simulink model "sampleModel337"  (R2021b)
settings: Solver=VariableStepAuto  StartTime=0.0  StopTime=10.0  RelTol=1e-3
undefined symbols (not defined in the file or in its folder): DiscIntNeverNeededParam, Newton, Raphson
libraries: simulink x14, slpidlib x1
settings Model: Creator=user  LastModifiedBy=user

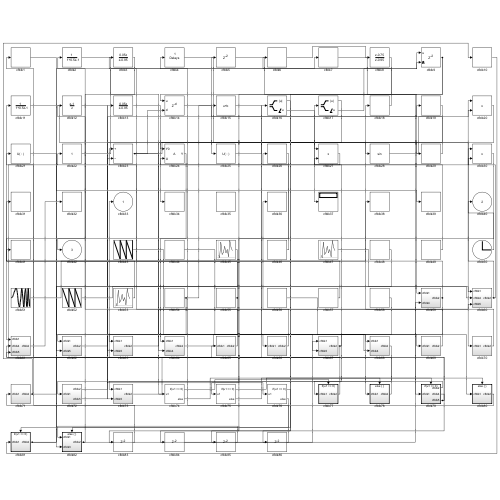
[thumbnail: Simulink's stored preview of the top-level diagram]
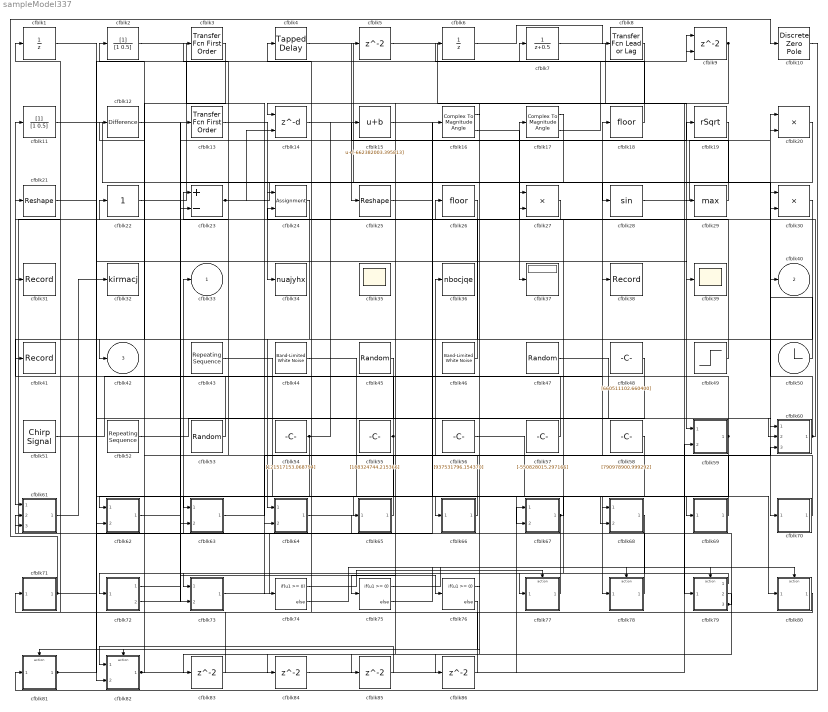
== system sampleModel337 ==
  cfblk1 : UnitDelay  HasFrameUpgradeWarning=on
  cfblk10 : DiscreteZeroPole  Poles=[0 0.5]  Gain=1
  cfblk11 : DiscreteFilter  SampleTime=1
  cfblk12 : simulink/Discrete/Difference  ICPrevInput=0.0  OutMin=[]  OutMax=[]  OutDataTypeStr=Inherit: Inherit via back propagation  OutDataType=fixdt(1, 16)  OutScaling=2^-10  DoSatur=off
  cfblk13 : simulink/Discrete/Transfer Fcn First Order  PoleZ=0.95  ICPrevOutput=0.0  DoSatur=off
  cfblk14 : Delay  DelayLengthSource=Input port  SampleTime=1
      settings: InputPortMap=u0,p1
  cfblk15 : Bias  Bias=[-662382003.395813]
  cfblk16 : ComplexToMagnitudeAngle
  cfblk17 : ComplexToMagnitudeAngle
  cfblk18 : Rounding
  cfblk19 : Sqrt  Operator=rSqrt  AlgorithmType=Newton-Raphson  SaturateOnIntegerOverflow=on
  cfblk2 : DiscreteFilter  SampleTime=1
  cfblk20 : Product
  cfblk21 : Reshape
  cfblk22 : simulink/Math Operations/Slider Gain  gain=1  low=0  high=2
  cfblk23 : Sum  Inputs=+-
  cfblk24 : Assignment  DiagnosticForDimensions=Warning  IndexOptions=Index vector (dialog)  Indices=1  OutputSizes=1
  cfblk25 : Reshape
  cfblk26 : Rounding
  cfblk27 : Product  Inputs=**
  cfblk28 : Trigonometry
  cfblk29 : MinMax  Function=max
  cfblk3 : simulink/Discrete/Transfer Fcn First Order  PoleZ=0.95  ICPrevOutput=0.0  DoSatur=off
  cfblk30 : Product  Inputs=**
  cfblk31 : Record  FileSettingsInternal="{\"entries\":[{\"content\":{\"excelSettings\":{\"content\":{},\"type\":\"Streamout.ExcelSettings\"}},\"type\":\"Streamout.FileSettingStorage\",\"uuid\":\"66267067-c99f-4175-8d2d-40c80f1adf8d\"}],\"packageUris\":[\"http://schema.mathworks.com/mf0/streamout_blocks/R2020a\"],\"version\":\"1.0\"}"  SignalsInternal="{\"entries\":[{\"content\":{\"signals\":[{\"content\":{\"blockPath\":[\"sampleModel337/cfblk31\"],\"channel\":[],\"dimensions\":[1],\"domain\":\"sampleModel337/cfblk31\",\"lineColor\":\"#fe330a\",\"plots\":[1],\"port\":1,\"sid\":[\"\"],\"signalID\":14199,\"signalName\":\"cfblk57\"},\"type\":\"RecordBlkView.Signal\",\"uuid\":\"3a15083e-2d8a-46d9-a8df-0416bb991a64\"}]},\"type\":\"RecordBlkView.InputSignals\",\"uuid\":\"83189cd0-23fa-40a2-b267-53570d34eaef\"}],\"packageUris\":[\"http://schema.mathworks.com/mf0/streamout_blocks/R2020a\"],\"version\":\"1.0\"}"  VisualizationBindings="{\"sparklinesplugin\":{\"info\":[{\"bindingParametersList\":[],\"subplotID\":1}]}}"
  cfblk32 : ToWorkspace  VariableName=kirmacj  SaveFormat=Timeseries  SampleTime=-1
  cfblk34 : ToWorkspace  VariableName=nuajyhx  SaveFormat=Timeseries  SampleTime=-1
  cfblk35 : Scope
      settings: Floating=on
  cfblk36 : ToWorkspace  VariableName=nbocjqe  SaveFormat=Timeseries  SampleTime=-1
  cfblk37 : Display
  cfblk38 : Record  FileSettingsInternal="{\"entries\":[{\"content\":{\"excelSettings\":{\"content\":{},\"type\":\"Streamout.ExcelSettings\"}},\"type\":\"Streamout.FileSettingStorage\",\"uuid\":\"2a3a7163-b390-43d8-9f29-9eb456848a90\"}],\"packageUris\":[\"http://schema.mathworks.com/mf0/streamout_blocks/R2020a\"],\"version\":\"1.0\"}"  SignalsInternal="{\"entries\":[{\"content\":{\"signals\":[{\"content\":{\"blockPath\":[\"sampleModel337/cfblk38\"],\"channel\":[],\"dimensions\":[1],\"domain\":\"sampleModel337/cfblk38\",\"lineColor\":\"#22b573\",\"plots\":[1],\"port\":1,\"sid\":[\"\"],\"signalID\":14203,\"signalName\":\"cfblk51\"},\"type\":\"RecordBlkView.Signal\",\"uuid\":\"ddd7f569-362b-4965-ba4b-a0f119b13426\"}]},\"type\":\"RecordBlkView.InputSignals\",\"uuid\":\"cd7c0851-9357-4c6c-955a-12bcfdba8bc9\"}],\"packageUris\":[\"http://schema.mathworks.com/mf0/streamout_blocks/R2020a\"],\"version\":\"1.0\"}"  VisualizationBindings="{\"sparklinesplugin\":{\"info\":[{\"bindingParametersList\":[],\"subplotID\":1}]}}"
  cfblk39 : Scope
  cfblk4 : simulink/Discrete/Tapped Delay  vinit=0.0  samptime=-1  NumDelays=1  DelayOrder=Oldest  includeCurrent=off
  cfblk41 : Record  FileSettingsInternal="{\"entries\":[{\"content\":{\"excelSettings\":{\"content\":{},\"type\":\"Streamout.ExcelSettings\"}},\"type\":\"Streamout.FileSettingStorage\",\"uuid\":\"26850afd-8027-4b58-a955-7d8a01ed87cd\"}],\"packageUris\":[\"http://schema.mathworks.com/mf0/streamout_blocks/R2020a\"],\"version\":\"1.0\"}"  SignalsInternal="{\"entries\":[{\"content\":{\"signals\":[{\"content\":{\"blockPath\":[\"sampleModel337/cfblk41\"],\"channel\":[],\"dimensions\":[1],\"domain\":\"sampleModel337/cfblk41\",\"lineColor\":\"#0072bd\",\"plots\":[1],\"port\":1,\"sid\":[\"\"],\"signalID\":14207,\"signalName\":\"cfblk53\"},\"type\":\"RecordBlkView.Signal\",\"uuid\":\"cd2cc7f3-c00a-4394-8ee3-9ab6e12422fb\"}]},\"type\":\"RecordBlkView.InputSignals\",\"uuid\":\"c4c34e3a-692d-469b-a801-c2dcdfd922a6\"}],\"packageUris\":[\"http://schema.mathworks.com/mf0/streamout_blocks/R2020a\"],\"version\":\"1.0\"}"  VisualizationBindings="{\"sparklinesplugin\":{\"info\":[{\"bindingParametersList\":[],\"subplotID\":1}]}}"
  cfblk43 : simulink/Sources/Repeating Sequence  rep_seq_t=[0 2]  rep_seq_y=[192165720.171164, -172473038.723980]
  cfblk44 : simulink/Sources/Band-Limited White Noise  Cov=[9425752500.272665]  Ts=0.1  seed=[1392653928.000000]
  cfblk45 : UniformRandomNumber  Minimum=[-7422839996.357573]  Maximum=[2193654231.156507]  Seed=[27006365.000000]  SampleTime=0.1
  cfblk46 : simulink/Sources/Band-Limited White Noise  Cov=[6685126925.213029]  Ts=0.1  seed=[6636375495.000000]
  cfblk47 : UniformRandomNumber  Minimum=[-5023507832.903557]  Maximum=[8728010214.788080]  Seed=[3871352.000000]  SampleTime=0.1
  cfblk48 : Constant  Value=[660511102.660400]  SampleTime=1
  cfblk49 : Step  Time=[24.000000]  Before=[-833293648.035745]  After=[-779564700.016699]  SampleTime=0
  cfblk{5,83..86} (5 alike) : Delay  SampleTime=1
  cfblk50 : Clock
  cfblk51 : simulink/Sources/Chirp Signal  f1=[227946711.193798]  T=[-292349557.338732]  f2=[-851109676.735082]
  cfblk52 : simulink/Sources/Repeating Sequence  rep_seq_t=[0 2]  rep_seq_y=[918778598.436416, 466082704.738296]
  cfblk53 : UniformRandomNumber  Minimum=[-5458441505.167678]  Maximum=[4282505821.018705]  Seed=[24483622.000000]  SampleTime=0.1
  cfblk54 : Constant  Value=[121517153.068794]  SampleTime=1
  cfblk55 : Constant  Value=[188324744.215366]  SampleTime=1
  cfblk56 : Constant  Value=[937531796.154370]  SampleTime=1
  cfblk57 : Constant  Value=[-550828015.297166]  SampleTime=1
  cfblk58 : Constant  Value=[790978900.999292]  SampleTime=1
  cfblk59 : Subsystem
  cfblk6 : UnitDelay  HasFrameUpgradeWarning=on
  cfblk60 : Subsystem
  cfblk61 : Subsystem
  cfblk62 : Subsystem
  cfblk63 : Subsystem
  cfblk64 : Subsystem
  cfblk65 : Subsystem
  cfblk66 : Subsystem
  cfblk67 : Subsystem
  cfblk68 : Subsystem
  cfblk69 : Subsystem
  cfblk7 : DiscreteTransferFcn  SampleTime=1
  cfblk70 : Subsystem
  cfblk71 : Subsystem
  cfblk72 : Subsystem
  cfblk73 : Subsystem
  cfblk74 : If  IfExpression=u1 >= 0  SampleTime=1
  cfblk75 : If  IfExpression=u1 >= 0  SampleTime=1
  cfblk76 : If  IfExpression=u1 >= 0  SampleTime=1
  cfblk77 : Subsystem  TreatAsAtomicUnit=on
  cfblk78 : Subsystem  TreatAsAtomicUnit=on
  cfblk79 : Subsystem  TreatAsAtomicUnit=on
  cfblk8 : simulink/Discrete/Transfer Fcn Lead or Lag  PoleZ=0.95  ZeroZ=0.75  ICPrevOutput=0.0  ICPrevInput=0.0  DoSatur=off
      settings: SourceProductBaseCode=SL
  cfblk80 : Subsystem  TreatAsAtomicUnit=on
  cfblk81 : Subsystem  TreatAsAtomicUnit=on
  cfblk82 : Subsystem  TreatAsAtomicUnit=on
  cfblk9 : Delay  ShowEnablePort=on  SampleTime=1
      settings: InputPortMap=u0,e6
  cfblk33 : Outport
  cfblk40 : Outport  Port=2
  cfblk42 : Outport  Port=3
  wires:
  cfblk61/1(cfblk2) -> cfblk32/1
  cfblk46/1 -> cfblk26/1
  cfblk70/1(cfblk2) -> cfblk18/1
  cfblk9/1 -> cfblk14/1, cfblk86/1
  cfblk66/1(cfblk2) -> cfblk36/1
  cfblk5/1 -> cfblk59/1(cfblk1)
  cfblk51/1 -> cfblk38/1
  cfblk55/1 -> cfblk62/1(cfblk1), cfblk3/1
  cfblk60/1(cfblk2) -> cfblk20/1, cfblk30/2
  cfblk17/1 -> cfblk34/1
  cfblk7/1 -> cfblk79/1(cfblk1)
  cfblk28/1 -> cfblk20/2
  cfblk67/1(cfblk2) -> cfblk22/1, cfblk27/2
  cfblk59/1(cfblk2) -> cfblk11/1, cfblk73/2(cfblk5)
  cfblk14/1 -> cfblk25/1
  cfblk23/1 -> cfblk29/1, cfblk14/2, cfblk67/2(cfblk5)
  cfblk26/1 -> cfblk64/1(cfblk1)
  cfblk24/1 -> cfblk61/1(cfblk1)
  cfblk21/1 -> cfblk39/1
  cfblk78/1(cfblk2) -> cfblk33/1
  cfblk54/1 -> cfblk63/1(cfblk1), cfblk15/1
  cfblk4/1 -> cfblk70/1(cfblk1)
  cfblk8/1 -> cfblk75/1
  cfblk62/1(cfblk2) -> cfblk19/1
  cfblk73/1(cfblk2) -> cfblk16/1
  cfblk11/1 -> cfblk28/1
  cfblk22/1 -> cfblk7/1
  cfblk82/1(cfblk2) -> cfblk2/1, cfblk59/2(cfblk4)
  cfblk72/1(cfblk2) -> cfblk13/1
  cfblk69/1(cfblk2) -> cfblk23/1
  cfblk44/1 -> cfblk80/1(cfblk1)
  cfblk81/1(cfblk2) -> cfblk30/1, cfblk9/2
  cfblk72/2(cfblk5) -> cfblk23/2
  cfblk56/1 -> cfblk78/1(cfblk1)
  cfblk43/1 -> cfblk69/1(cfblk1)
  cfblk80/1(cfblk2) -> cfblk71/1(cfblk1)
  cfblk57/1 -> cfblk31/1
  cfblk48/1 -> cfblk82/2(cfblk3)
  cfblk16/2 -> cfblk37/1
  cfblk68/1(cfblk2) -> cfblk72/1(cfblk1)
  cfblk71/1(cfblk2) -> cfblk10/1, cfblk65/1(cfblk1)
  cfblk53/1 -> cfblk41/1
  cfblk19/1 -> cfblk63/2(cfblk5)
  cfblk65/1(cfblk2) -> cfblk12/1
  cfblk3/1 -> cfblk42/1
  cfblk47/1 -> cfblk60/1(cfblk1)
  cfblk77/1(cfblk2) -> cfblk21/1
  cfblk49/1 -> cfblk17/1
  cfblk13/1 -> cfblk24/1
  cfblk20/1 -> cfblk64/2(cfblk4)
  cfblk12/1 -> cfblk76/1
  cfblk10/1 -> cfblk81/1(cfblk1)
  cfblk1/1 -> cfblk68/1(cfblk1)
  cfblk64/1(cfblk2) -> cfblk66/1(cfblk1)
  cfblk50/1 -> cfblk40/1
  cfblk27/1 -> cfblk24/2
  cfblk45/1 -> cfblk62/2(cfblk5)
  cfblk15/1 -> cfblk68/2(cfblk4)
  cfblk25/1 -> cfblk27/1
  cfblk6/1 -> cfblk8/1
  cfblk18/1 -> cfblk6/1
  cfblk2/1 -> cfblk74/1
  cfblk52/1 -> cfblk60/2(cfblk4)
  cfblk63/1(cfblk2) -> cfblk60/3(cfblk5)
  cfblk29/1 -> cfblk5/1
  cfblk79/1(cfblk2) -> cfblk73/1(cfblk1)
  cfblk79/3(cfblk5) -> cfblk61/2(cfblk4), cfblk61/3(cfblk5)
  cfblk58/1 -> cfblk77/1(cfblk1)
  cfblk17/2 -> cfblk9/1
  cfblk74/1 -> cfblk77/Action
  cfblk74/2 -> cfblk78/Action
  cfblk75/1 -> cfblk79/Action
  cfblk75/2 -> cfblk80/Action
  cfblk76/1 -> cfblk81/Action
  cfblk76/2 -> cfblk82/Action
  cfblk16/1 -> cfblk83/1
  cfblk83/1 -> cfblk1/1
  cfblk79/2(cfblk4) -> cfblk84/1
  cfblk84/1 -> cfblk67/1(cfblk1)
  cfblk30/1 -> cfblk85/1
  cfblk85/1 -> cfblk82/1(cfblk1)
  cfblk86/1 -> cfblk4/1

== system sampleModel337/cfblk59 ==
  cfblk1 : Inport
  cfblk4 : Inport  Port=2
  cfblk3 : Constant  Value=[731305809.707664]  SampleTime=1
  cfblk2 : Outport
  wires:
  cfblk1/1 -> cfblk2/1

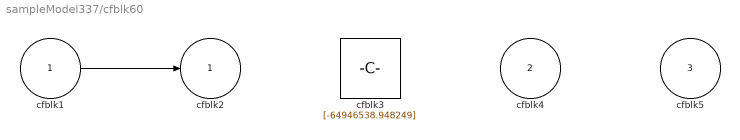
== system sampleModel337/cfblk60 ==
  cfblk1 : Inport
  cfblk4 : Inport  Port=2
  cfblk5 : Inport  Port=3
  cfblk3 : Constant  Value=[-64946538.948249]  SampleTime=1
  cfblk2 : Outport
  wires:
  cfblk1/1 -> cfblk2/1

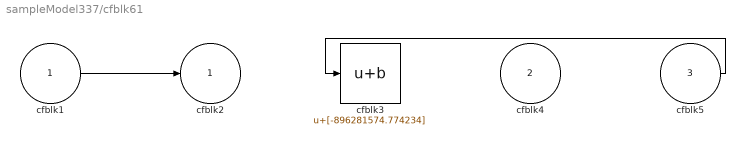
== system sampleModel337/cfblk61 ==
  cfblk1 : Inport
  cfblk4 : Inport  Port=2
  cfblk5 : Inport  Port=3
  cfblk3 : Bias  Bias=[-896281574.774234]
  cfblk2 : Outport
  wires:
  cfblk1/1 -> cfblk2/1
  cfblk5/1 -> cfblk3/1

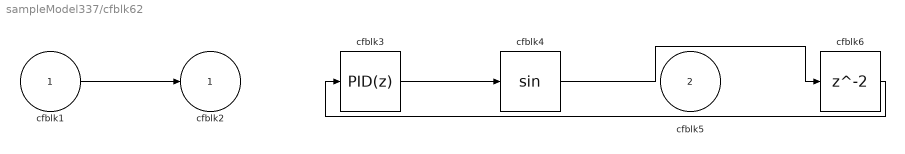
== system sampleModel337/cfblk62 ==
  cfblk1 : Inport
  cfblk5 : Inport  Port=2
  cfblk3 : slpidlib/PID Controller  Controller=PID  Form=Parallel  TimeDomain=Discrete-time  UseExternalTs=off  SampleTime=1  IntegratorMethod=Forward Euler  FilterMethod=Forward Euler  ControllerParametersSource=internal  P=1  I=1  D=0  UseFilter=on  N=100  TunerSelectOption=Transfer Function Based (PID Tuner App)  InitialConditionSource=internal  InitialConditionForIntegrator=0  InitialConditionForFilter=0  DifferentiatorICPrevScaledInput=0  ExternalReset=none  TrackingMode=off  Kt=1  LimitOutput=off  SatLimitsSource=internal  UpperSaturationLimit=inf  LowerSaturationLimit=-inf  LinearizeAsGain=off  AntiWindupMode=none  Kb=1  POutMin=[]  POutMax=[]  IOutMin=[]  IOutMax=[]  DOutMin=[]  DOutMax=[]  NOutMin=[]  NOutMax=[]  SumOutMin=[]  SumOutMax=[]  SaturationOutMin=[]  SaturationOutMax=[]  PParamMin=[]  PParamMax=[]  IParamMin=[]  IParamMax=[]  DParamMin=[]  DParamMax=[]  NParamMin=[]  NParamMax=[]  KbParamMin=[]  KbParamMax=[]  KtParamMin=[]  KtParamMax=[]  KbOutMin=[]  KbOutMax=[]  KtOutMin=[]  KtOutMax=[]  IntegratorOutMin=[]  IntegratorOutMax=[]  FilterOutMin=[]  FilterOutMax=[]  SumI1OutMin=[]  SumI1OutMax=[]  SumI2OutMin=[]  SumI2OutMax=[]  SumI3OutMin=[]  SumI3OutMax=[]  SumI4OutMin=[]  SumI4OutMax=[]  SumDOutMin=[]  SumDOutMax=[]  DifferentiatorOutMin=[]  DifferentiatorOutMax=[]  FilterDiffOutCoefMin=[]  FilterDiffOutCoefMax=[]  ReciprocalOutMin=[]  ReciprocalOutMax=[]  SumDenOutMin=[]  SumDenOutMax=[]  SumNumOutMin=[]  SumNumOutMax=[]  DivideOutMin=[]  DivideOutMax=[]  UdiffTsProdOutMin=[]  UdiffTsProdOutMax=[]  NTsProdOutMin=[]  NTsProdOutMax=[]  UintegralTsProdOutMin=[]  UintegralTsProdOutMax=[]  UngainTsProdOutMin=[]  UngainTsProdOutMax=[]  IntegratorContinuousStateAttributes=''  IntegratorStateMustResolveToSignalObject=off  IntegratorRTWStateStorageClass=Auto  FilterContinuousStateAttributes=''  FilterStateMustResolveToSignalObject=off  FilterRTWStateStorageClass=Auto  ParallelPVariant=InternalParameters  IdealPVariant=Disabled  IVariant=InternalParameters  DVariant=InternalParameters  IntegratorVariant=Discrete  SatVariant=Disabled  AWVariant=Passthrough  PCopyVariant=Disabled  TRVariant=Disabled  FdbkBlocksVariant=Forward  IdealPFdbkVariant=Disabled  SatFdbkVariant=Disabled  DerivativeFilterVariant=ForwardEulerFilter  NVariant=InternalParameters  NCopyVariant=Disabled  FilterICVariant=InternalICsFilter  IntegratorICVariant=InternalICs  ExternalResetVariant=Disabled  TRSumVariant=Passthrough  SumFdbkVariant=Disabled  SumVariant=Sum_PID  TsampFilterVariant=InternalTs  TsampNgainVariant=Passthrough  TsampIntegralVariant=Passthrough  ExternalSaturationOutDataTypeStr=Inherit: Same as second input
  cfblk4 : Trigonometry
  cfblk6 : Delay  SampleTime=1
  cfblk2 : Outport
  wires:
  cfblk1/1 -> cfblk2/1
  cfblk3/1 -> cfblk4/1
  cfblk4/1 -> cfblk6/1
  cfblk6/1 -> cfblk3/1

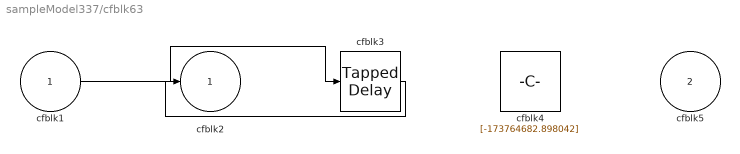
== system sampleModel337/cfblk63 ==
  cfblk1 : Inport
  cfblk5 : Inport  Port=2
  cfblk3 : simulink/Discrete/Tapped Delay  vinit=0.0  samptime=-1  NumDelays=1  DelayOrder=Oldest  includeCurrent=off
  cfblk4 : Constant  Value=[-173764682.898042]  SampleTime=1
  cfblk2 : Outport
  wires:
  cfblk1/1 -> cfblk3/1
  cfblk3/1 -> cfblk2/1

== system sampleModel337/cfblk64 ==
  cfblk1 : Inport
  cfblk4 : Inport  Port=2
  cfblk3 : Product  Inputs=*
  cfblk2 : Outport
  wires:
  cfblk1/1 -> cfblk3/1
  cfblk3/1 -> cfblk2/1

== system sampleModel337/cfblk65 ==
  cfblk1 : Inport
  cfblk3 : Sum  Inputs=+-
  cfblk4 : Constant  Value=[-405894164.948461]  SampleTime=1
  cfblk2 : Outport
  wires:
  cfblk4/1 -> cfblk2/1, cfblk3/2
  cfblk1/1 -> cfblk3/1

== system sampleModel337/cfblk66 ==
  cfblk1 : Inport
  cfblk3 : Delay  ShowEnablePort=on  SampleTime=1
      settings: InputPortMap=u0,e6
  cfblk2 : Outport
  wires:
  cfblk1/1 -> cfblk3/1, cfblk3/2
  cfblk3/1 -> cfblk2/1

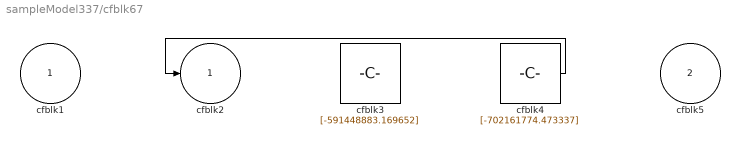
== system sampleModel337/cfblk67 ==
  cfblk1 : Inport
  cfblk5 : Inport  Port=2
  cfblk3 : Constant  Value=[-591448883.169652]  SampleTime=1
  cfblk4 : Constant  Value=[-702161774.473337]  SampleTime=1
  cfblk2 : Outport
  wires:
  cfblk4/1 -> cfblk2/1

== system sampleModel337/cfblk68 ==
  cfblk1 : Inport
  cfblk4 : Inport  Port=2
  cfblk3 : Sin  TimeSource=Use external signal  SampleTime=0
  cfblk2 : Outport
  wires:
  cfblk4/1 -> cfblk3/1
  cfblk1/1 -> cfblk2/1

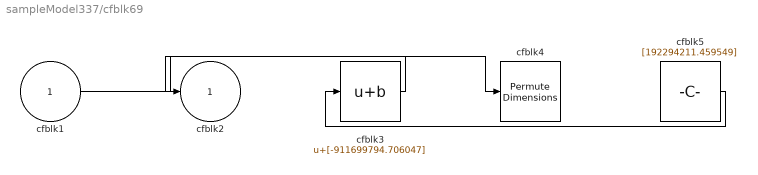
== system sampleModel337/cfblk69 ==
  cfblk1 : Inport
  cfblk3 : Bias  Bias=[-911699794.706047]
  cfblk4 : PermuteDimensions
  cfblk5 : Constant  Value=[192294211.459549]  SampleTime=1
  cfblk2 : Outport
  wires:
  cfblk1/1 -> cfblk4/1
  cfblk5/1 -> cfblk3/1
  cfblk3/1 -> cfblk2/1

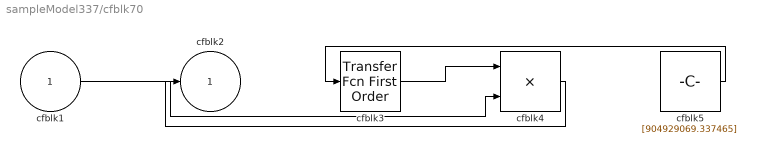
== system sampleModel337/cfblk70 ==
  cfblk1 : Inport
  cfblk3 : simulink/Discrete/Transfer Fcn First Order  PoleZ=0.95  ICPrevOutput=0.0  DoSatur=off
  cfblk4 : Product
  cfblk5 : Constant  Value=[904929069.337465]  SampleTime=1
  cfblk2 : Outport
  wires:
  cfblk3/1 -> cfblk4/1
  cfblk1/1 -> cfblk4/2
  cfblk5/1 -> cfblk3/1
  cfblk4/1 -> cfblk2/1

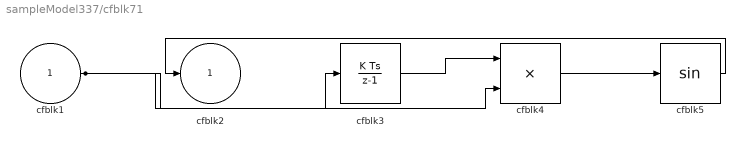
== system sampleModel337/cfblk71 ==
  cfblk1 : Inport
  cfblk3 : DiscreteIntegrator  ICPrevOutput=DiscIntNeverNeededParam  ICPrevScaledInput=DiscIntNeverNeededParam
  cfblk4 : Product  Inputs=**
  cfblk5 : Trigonometry
  cfblk2 : Outport
  wires:
  cfblk5/1 -> cfblk2/1
  cfblk1/1 -> cfblk3/1, cfblk4/2
  cfblk3/1 -> cfblk4/1
  cfblk4/1 -> cfblk5/1

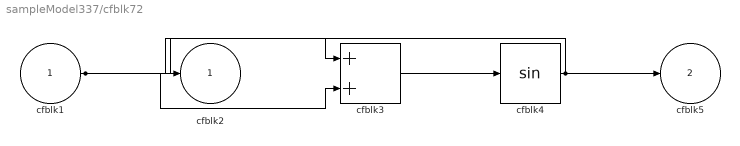
== system sampleModel337/cfblk72 ==
  cfblk1 : Inport
  cfblk3 : Sum
  cfblk4 : Trigonometry
  cfblk2 : Outport
  cfblk5 : Outport  Port=2
  wires:
  cfblk3/1 -> cfblk4/1
  cfblk4/1 -> cfblk5/1, cfblk2/1
  cfblk1/1 -> cfblk3/1, cfblk3/2

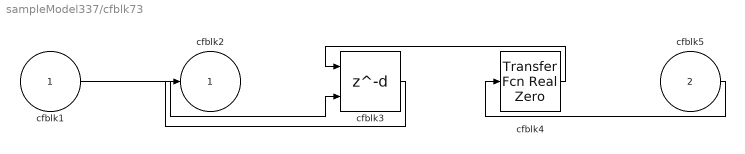
== system sampleModel337/cfblk73 ==
  cfblk1 : Inport
  cfblk5 : Inport  Port=2
  cfblk3 : Delay  DelayLengthSource=Input port  SampleTime=1
      settings: InputPortMap=u0,p1
  cfblk4 : simulink/Discrete/Transfer Fcn Real Zero  ZeroZ=0.75  ICPrevInput=0.0  DoSatur=off
      settings: SourceProductBaseCode=SL
  cfblk2 : Outport
  wires:
  cfblk4/1 -> cfblk3/1
  cfblk5/1 -> cfblk4/1
  cfblk1/1 -> cfblk3/2
  cfblk3/1 -> cfblk2/1

== system sampleModel337/cfblk77 ==
  cfblk1 : Inport
  Action Port : ActionPort  ActionPortLabel=if(u1 >= 0)
  cfblk3 : ComplexToMagnitudeAngle
  cfblk2 : Outport
  wires:
  cfblk1/1 -> cfblk2/1, cfblk3/1

== system sampleModel337/cfblk78 ==
  cfblk1 : Inport
  Action Port : ActionPort  ActionPortLabel=else
  cfblk3 : Delay  DelayLengthSource=Input port
      settings: InputPortMap=u0,p1
  cfblk2 : Outport
  wires:
  cfblk1/1 -> cfblk3/1, cfblk3/2
  cfblk3/1 -> cfblk2/1

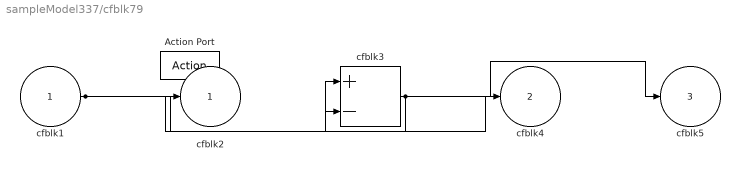
== system sampleModel337/cfblk79 ==
  cfblk1 : Inport
  Action Port : ActionPort  ActionPortLabel=if(u1 >= 0)
  cfblk3 : Sum  Inputs=+-
  cfblk2 : Outport
  cfblk4 : Outport  Port=2
  cfblk5 : Outport  Port=3
  wires:
  cfblk1/1 -> cfblk3/1, cfblk3/2, cfblk4/1
  cfblk3/1 -> cfblk5/1, cfblk2/1

== system sampleModel337/cfblk80 ==
  cfblk1 : Inport
  Action Port : ActionPort  ActionPortLabel=else
  cfblk3 : Gain  Gain=[-544598460.362439]
  cfblk2 : Outport
  wires:
  cfblk1/1 -> cfblk2/1, cfblk3/1

== system sampleModel337/cfblk81 ==
  cfblk1 : Inport
  Action Port : ActionPort  ActionPortLabel=if(u1 >= 0)
  cfblk3 : Constant  Value=[-248883315.456549]  SampleTime=1
  cfblk2 : Outport
  wires:
  cfblk1/1 -> cfblk2/1

== system sampleModel337/cfblk82 ==
  cfblk1 : Inport
  cfblk3 : Inport  Port=2
  Action Port : ActionPort  ActionPortLabel=else
  cfblk2 : Outport
  wires:
  cfblk3/1 -> cfblk2/1
